simulink model "c_lab4sim_b"  (R2020b)
settings: Solver=VariableStepAuto  StartTime=0.0  StopTime=10.0  RelTol=1e-3
settings Model: Creator=musa oğural  LastModifiedBy=musa oğural

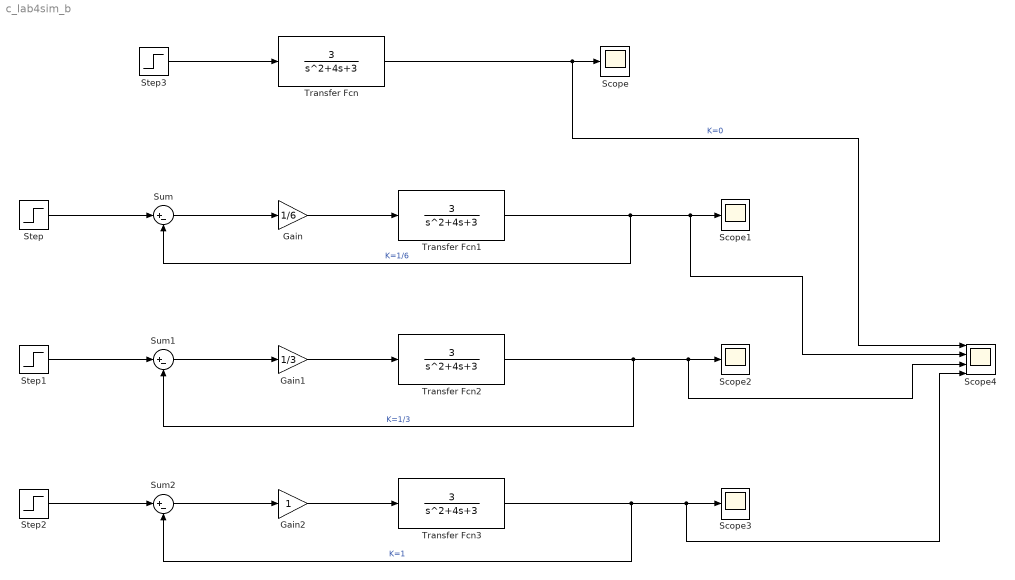
== system c_lab4sim_b ==
  Gain : Gain  Gain=1/6
  Gain1 : Gain  Gain=1/3
  Gain2 : Gain
  Scope{,1..3} (4 alike) : Scope
  Scope4 : Scope  NumInputPorts=4
  Step{,1..3} (4 alike) : Step  Time=0  SampleTime=0
  Sum : Sum  Inputs=|+-
  Sum1 : Sum  Inputs=|+-
  Sum2 : Sum  Inputs=|+-
  Transfer Fcn{,1..3} (4 alike) : TransferFcn  Numerator=[3]  Denominator=[1 4 3]
  wires:
  Step3/1 -> Transfer Fcn/1
  Transfer Fcn/1 -> Scope4/1, Scope/1  "K=0"
  Step/1 -> Sum/1
  Sum/1 -> Gain/1
  Gain/1 -> Transfer Fcn1/1
  Step1/1 -> Sum1/1
  Sum1/1 -> Gain1/1
  Gain1/1 -> Transfer Fcn2/1
  Step2/1 -> Sum2/1
  Sum2/1 -> Gain2/1
  Gain2/1 -> Transfer Fcn3/1
  Transfer Fcn3/1 -> Sum2/2, Scope4/4, Scope3/1  "K=1"
  Transfer Fcn1/1 -> Sum/2, Scope4/2, Scope1/1  "K=1/6"
  Transfer Fcn2/1 -> Sum1/2, Scope4/3, Scope2/1  "K=1/3"
